simulink model "MRAC_Thermal_System"  (R2025b)
settings: Solver=VariableStepAuto  StartTime=0.0  StopTime=2e07  RelTol=1e-3
InitFcn:
  | a=1;
  | b=2;
  | C=(5+a+b)*1000;
  | K=20*(a+b+1);
  | b_p=1/C;
  | a_p=K/C;
  | T_constant_p=1/a_p;
  | T_constant_m=0.5*T_constant_p;
  | a_m=1/T_constant_m;
  | b_m = a_m;
  | Theta1_opt = b_m/b_p;
  | Theta2_opt=(-a_m+a_p)/-b_p;
  | Theta3_opt=a_p/b_p;
model workspace (MAT data in the model file):
  Sig = Simulink.Signal
  Sig.Dimensions = -1
  Sig.DimensionsMode = 'auto'
  Sig.Complexity = 'auto'
  Sig.SampleTime = -1
  Sig.SamplingMode = 'auto'
  Sig.DataType = 'auto'
  U_max = 2500
  U_min = -1200
  a = 1
  b = 2
  gamma = 40
settings Model: Creator=Ahmed  LastModifiedBy=Ahmed

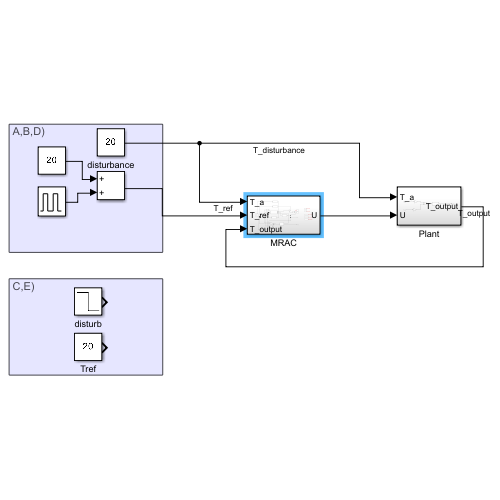
[thumbnail: Simulink's stored preview of the top-level diagram]
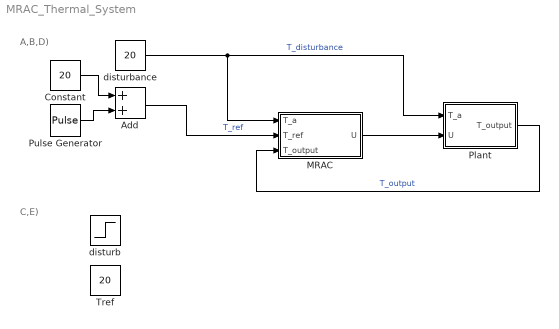
== system MRAC_Thermal_System ==
  note: A,B,D)
  note: C,E)
  Add : Sum
  Constant : Constant  Value=20
  MRAC : Subsystem
  Plant : Subsystem
  Pulse Generator : DiscretePulseGenerator  PulseType=Time based  Amplitude=10  Period=10000  PulseWidth=50
  Tref : Constant  Value=20
  disturb : Step  Time=200  Before=20  After=15  SampleTime=0
  disturbance : Constant  Value=20
  wires:
  Add/1 -> MRAC/2(T_ref)  "T_ref"
  MRAC/1(U) -> Plant/2(U)
  disturbance/1 -> MRAC/1(T_a), Plant/1(T_a)  "T_disturbance"
  Plant/1(T_output) -> MRAC/3(T_output)  "T_output"
  Constant/1 -> Add/1
  Pulse Generator/1 -> Add/2

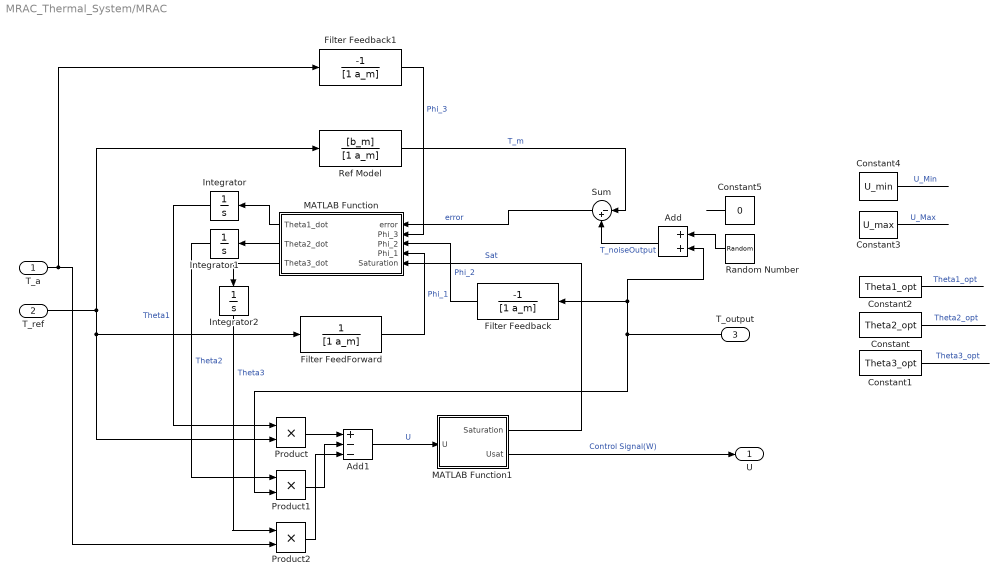
== system MRAC_Thermal_System/MRAC ==
  T_a : Inport
  T_ref : Inport  Port=2
  T_output : Inport  Port=3
  Add : Sum
  Add1 : Sum  Inputs=+--
  Constant : Constant  Value=Theta2_opt
  Constant1 : Constant  Value=Theta3_opt
  Constant2 : Constant  Value=Theta1_opt
  Constant3 : Constant  Value=U_max
  Constant4 : Constant  Value=U_min
  Constant5 : Constant  Value=0
  Filter FeedForward : TransferFcn  Denominator=[1 a_m]
  Filter Feedback : TransferFcn  Numerator=[-1]  Denominator=[1 a_m]
  Filter Feedback1 : TransferFcn  Numerator=[-1]  Denominator=[1 a_m]
  Integrator : Integrator  InitialCondition=0 %Theta1_opt
  Integrator1 : Integrator  InitialCondition=0%Theta2_opt
  Integrator2 : Integrator  InitialCondition=0%Theta3_opt
  MATLAB Function : MATLAB Function  TreatAsAtomicUnit=on
  MATLAB Function1 : MATLAB Function  TreatAsAtomicUnit=on
  Product : Product
  Product1 : Product
  Product2 : Product
  Random Number : RandomNumber  Variance=sqrt(0.5)
  Ref Model : TransferFcn  Numerator=[b_m]  Denominator=[1 a_m]
  Sum : Sum  Inputs=|-+
  U : Outport
  wires:
  Add1/1 -> MATLAB Function1/1(U)  "U"
  Filter FeedForward/1 -> MATLAB Function/4(Phi_1)  "Phi_1"
  MATLAB Function/2(Theta2_dot) -> Integrator1/1
  T_output/1 -> Add/2, Filter Feedback/1, Product1/2
  MATLAB Function/1(Theta1_dot) -> Integrator/1
  T_ref/1 -> Product/2, Filter FeedForward/1, Ref Model/1
  Ref Model/1 -> Sum/1  "T_m"
  Product1/1 -> Add1/2
  Product/1 -> Add1/1
  Sum/1 -> MATLAB Function/1(error)  "error"
  Integrator1/1 -> Product1/1  "Theta2"
  Integrator/1 -> Product/1  "Theta1"
  Filter Feedback/1 -> MATLAB Function/3(Phi_2)  "Phi_2"
  MATLAB Function1/2(Usat) -> U/1  "Control Signal(W)"
  Product2/1 -> Add1/3
  T_a/1 -> Filter Feedback1/1, Product2/2
  Filter Feedback1/1 -> MATLAB Function/2(Phi_3)  "Phi_3"
  MATLAB Function/3(Theta3_dot) -> Integrator2/1
  Integrator2/1 -> Product2/1  "Theta3"
  Constant2/1 -> ?  "Theta1_opt"
  Constant/1 -> ?  "Theta2_opt"
  Constant1/1 -> ?  "Theta3_opt"
  Constant3/1 -> ?  "U_Max"
  Constant4/1 -> ?  "U_Min"
  MATLAB Function1/1(Saturation) -> MATLAB Function/5(Saturation)  "Sat"
  Random Number/1 -> Add/1
  Add/1 -> Sum/2  "T_noiseOutput"
  Constant5/1 -> ?

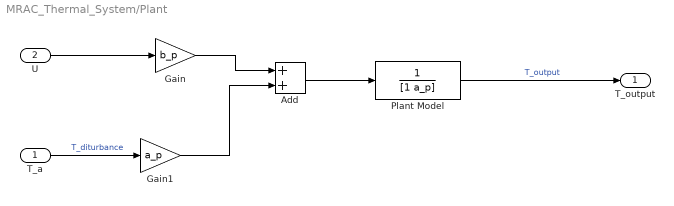
== system MRAC_Thermal_System/Plant ==
  T_a : Inport
  U : Inport  Port=2
  Add : Sum
  Gain : Gain  Gain=b_p
  Gain1 : Gain  Gain=a_p
  Plant Model : TransferFcn  Denominator=[1 a_p]
  T_output : Outport
  wires:
  Gain1/1 -> Add/2
  Add/1 -> Plant Model/1
  T_a/1 -> Gain1/1  "T_diturbance"
  Gain/1 -> Add/1
  U/1 -> Gain/1
  Plant Model/1 -> T_output/1  "T_output"

== matlab function MRAC_Thermal_System/MRAC/MATLAB Function1 ==
  data: U input; Saturation output; Usat output; U_max parameter; U_min parameter
function [Saturation,Usat] = fcn(U,U_max, U_min)

if U>=U_max
    Usat=U_max;
    Saturation = true;
elseif U<=U_min
    Usat=U_min;
    Saturation = true;
else
    Usat=U;
    Saturation=false;
end

== matlab function MRAC_Thermal_System/MRAC/MATLAB Function ==
  data: error input; Phi_3 input; Phi_2 input; Phi_1 input; Theta1_dot output; Theta2_dot output; gamma parameter; Theta3_dot output; Saturation input
function [Theta1_dot , Theta2_dot, Theta3_dot]= fcn(error ,Phi_3,Phi_2,Phi_1, gamma, Saturation)

alpha =0.001;

if Saturation==false
    Theta1_dot = ( -1*gamma*error*Phi_1)/(alpha+Phi_1^2+Phi_2^2+Phi_3^2);
    Theta2_dot = ( -1*gamma*error*Phi_2)/(alpha+Phi_1^2+Phi_2^2+Phi_3^2);
    Theta3_dot = ( -1*gamma*error*Phi_3)/(alpha+Phi_1^2+Phi_2^2+Phi_3^2);
else
    Theta1_dot =0;
    Theta2_dot =0;
    Theta3_dot =0;
end
